simulink model "TLNWithUnrealTestBench"  (R2022b)
settings: Solver=VariableStepAuto  StartTime=0.0  StopTime=scenario.StopTime  FixedStep=0.001  RelTol=1e-8  EnableMultiTasking=on
PostLoadFcn:
  | helperSLTrafficLightNegotiationWithUnrealSetup
values from neighbouring files (symbols this model uses):
  vehSim3D = repmat(         struct(             'Length', 0,             'RearOverhang', 0,             'InitialPos',[0 0 0],             'InitialRot',[0 0 0]),         numVehicles,1)    [helperSLVisionVehicleDetectorSetup.m]
undefined symbols (not defined in the file or in its folder): Curvature, CurvatureDerivative, driving, gray, HeadingAngle, intersectionInfo, LateralOffset, Left, M, matlabshared, N, referencePathInfo, Right, setVelocity, strel, Strength, trafficLightConfig, Ts
libraries: drivingscenarioandsensors x7, visionsinks x4, visiontextngfix x3, sim3dautolib x3, sim3dlib x2, visionstatistics x1, visionmorphops x1, sim3dcameralib x1, helperTrafficLightControllerLib x1, trackingutilitieslib x1, drivinglib x1
CloseFcn:
  | helperSLTrafficLightNegotiationWithUnrealCleanUp
settings Model: Creator=The MathWorks, Inc.  LastModifiedBy=Administrator
settings SolverCC: ZeroCrossAlgorithm=Adaptive  AlgebraicLoopSolver=TrustRegion  PositivePriorityOrder=on  AutoInsertRateTranBlk=on  InsertRTBMode=Always  DecoupledContinuousIntegration=on  MinimalZcImpactIntegration=on  MaxZcPerStep=1
settings DataIOCC: SaveOutput=off  SaveTime=off  ReturnWorkspaceOutputs=off
settings OptimizationCC: DefaultParameterBehavior=Inlined  EnhancedBackFolding=on  PassReuseOutputArgsAs=Individual arguments  ZeroExternalMemoryAtStartup=off  ZeroInternalMemoryAtStartup=off  OptimizeBlockOrder=speed  DifferentSizesBufferReuse=on  OptimizationCustomize=off  EfficientTunableParamExpr=on
settings DebuggingCC: MaskedZcDiagnostic=none  IgnoredZcDiagnostic=none  ParameterPrecisionLossMsg=none  ParameterTunabilityLossMsg=error  UnconnectedInputMsg=warning  UnconnectedOutputMsg=warning  UnconnectedLineMsg=warning  PregeneratedLibrarySubsystemCodeDiagnostic=none  SFMachineParentedDataDiag=warning  ArithmeticOperatorsInVariantConditions=warning
settings HardwareCC: ProdLongLongMode=on
settings ModelReferenceCC: EnableRefExpFcnMdlSchedulingChecks=on
settings SFSimCC: SimUseLocalCustomCode=off  MATLABDynamicMemAlloc=off
settings RTWCC: Description=Embedded Coder  SystemTargetFile=ert.tlc  TemplateMakefile=ert_default_tmf  GenerateReport=on  RTWUseLocalCustomCode=off  LaunchReport=on  DLArmComputeVersion=19.05
settings CodeAppCC: ForceParamTrailComments=on  IgnoreCustomStorageClasses=off  OperatorAnnotations=on  SimulinkDataObjDesc=on  SFDataObjDesc=on  InsertBlockDesc=on
settings ERTTargetCC: TargetLangStandard=C99 (ISO)  GenerateSampleERTMain=on  InlinedParameterPlacement=NonHierarchical  ERTCustomFileTemplate=example_file_process.tlc
settings ConfigComp: CovScope=ReferencedModels  CovIncludeTopModel=off

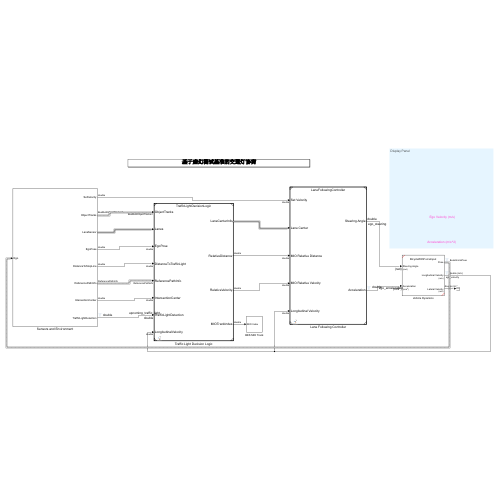
[thumbnail: Simulink's stored preview of the top-level diagram]
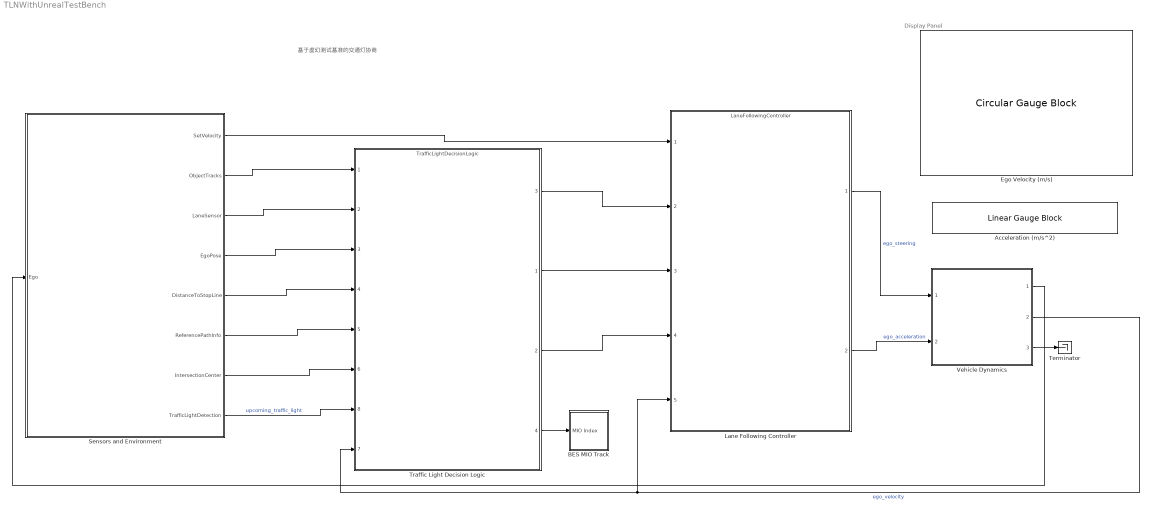
== system TLNWithUnrealTestBench ==
  note: 基于虚幻测试基准的交通灯协商
  note: Display Panel
  Acceleration (m/s^2) : LinearGaugeBlock  LabelPosition=Hide  ScaleMin=-6  ScaleMax=6
  BES MIO Track : Subsystem
  Ego Velocity (m/s) : CircularGaugeBlock  LabelPosition=Hide  ScaleMax=50
  Lane Following Controller : ModelReference  ModelNameDialog=LaneFollowingController.slx  SimulationMode=Normal  ModelReferenceVersion=6.0
  Sensors and Environment : Subsystem
  Terminator : Terminator
  Traffic Light Decision Logic : ModelReference  ModelNameDialog=TrafficLightDecisionLogic  SimulationMode=Normal  ModelReferenceVersion=5.0
      settings: PortSchema="{\"entries\":[{\"content\":{\"sides\":[{\"content\":{\"connectorIds\":[\"In1\",\"In2\",\"In3\",\"In4\",\"In5\",\"In6\",\"In8\",\"In7\"]},\"type\":\"ConnectorPlacement.EquallySpacedRectSide\",\"uuid\":\"80441088-7f88-498e-bd57-56a9591db5ab\"},{\"content\":{\"connectorIds\":[\"Out3\",\"Out1\",\"Out2\",\"Out4\"],\"side\":\"RIGHT\"},\"type\":\"ConnectorPlacement.EquallySpacedRectSide\",\"uuid\":\"71bac071-b53b-4fb3-8fe7-17db6e81a6fe\"},{\"content\":{\"connectorIds\":[],\"side\":\"TOP\"},\"type\":\"ConnectorPlacement.EquallySpacedRectSide\",\"uuid\":\"95fcddf4-1608-4cb5-a6ec-8633d9712dcc\"},{\"content\":{\"connectorIds\":[],\"side\":\"HIDDEN\"},\"type\":\"ConnectorPlacement.EquallySpacedRectSide\",\"uuid\":\"8d5e9fdd-dbcd-4e58-97a7-7da238f3d39d\"}]},\"type\":\"ConnectorPlacement.EquallySpacedConnector\",\"uuid\":\"78ce1c2f-8a23-470e-877e-968badbfaf17\"}],\"packageUris\":[\"http://schema.mathworks.com/mf0/Connector/R2020b\"],\"version\":\"1.0\"}"
  Vehicle Dynamics : Subsystem  ReferencedSubsystem=BicycleWithForceInput
  wires:
  Sensors and Environment/2(ObjectTracks) -> Traffic Light Decision Logic/1
  Sensors and Environment/1(SetVelocity) -> Lane Following Controller/1
  Sensors and Environment/8(TrafficLightDetection) -> Traffic Light Decision Logic/8  "upcoming_traffic_light"
  Vehicle Dynamics/1 -> Sensors and Environment/1(Ego)
  Sensors and Environment/4(EgoPose) -> Traffic Light Decision Logic/3
  Sensors and Environment/3(LaneSensor) -> Traffic Light Decision Logic/2
  Sensors and Environment/5(DistanceToStopLine) -> Traffic Light Decision Logic/4
  Sensors and Environment/6(ReferencePathInfo) -> Traffic Light Decision Logic/5
  Sensors and Environment/7(IntersectionCenter) -> Traffic Light Decision Logic/6
  Lane Following Controller/1 -> Vehicle Dynamics/1  "ego_steering"
  Lane Following Controller/2 -> Vehicle Dynamics/2  "ego_acceleration"
  Traffic Light Decision Logic/3 -> Lane Following Controller/2
  Traffic Light Decision Logic/1 -> Lane Following Controller/3
  Traffic Light Decision Logic/2 -> Lane Following Controller/4
  Traffic Light Decision Logic/4 -> BES MIO Track/1(MIO Index)
  Vehicle Dynamics/2 -> Lane Following Controller/5, Traffic Light Decision Logic/7  "ego_velocity"
  Vehicle Dynamics/3 -> Terminator/1

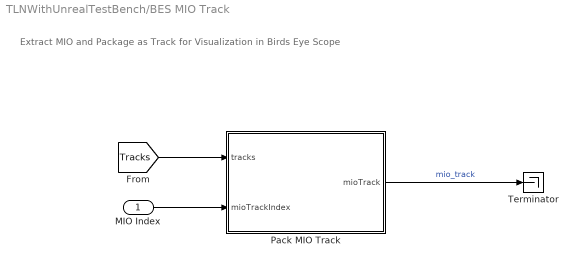
== system TLNWithUnrealTestBench/BES MIO Track ==
  note: Extract MIO and Package as Track for Visualization in Birds Eye Scope
  MIO Index : Inport
  Pack MIO Track : MATLAB Function  TreatAsAtomicUnit=on
  Terminator : Terminator
  wires:
  MIO Index/1 -> Pack MIO Track/2(mioTrackIndex)
  [Tracks] -> Pack MIO Track/1(tracks)
  Pack MIO Track/1(mioTrack) -> Terminator/1  "mio_track"

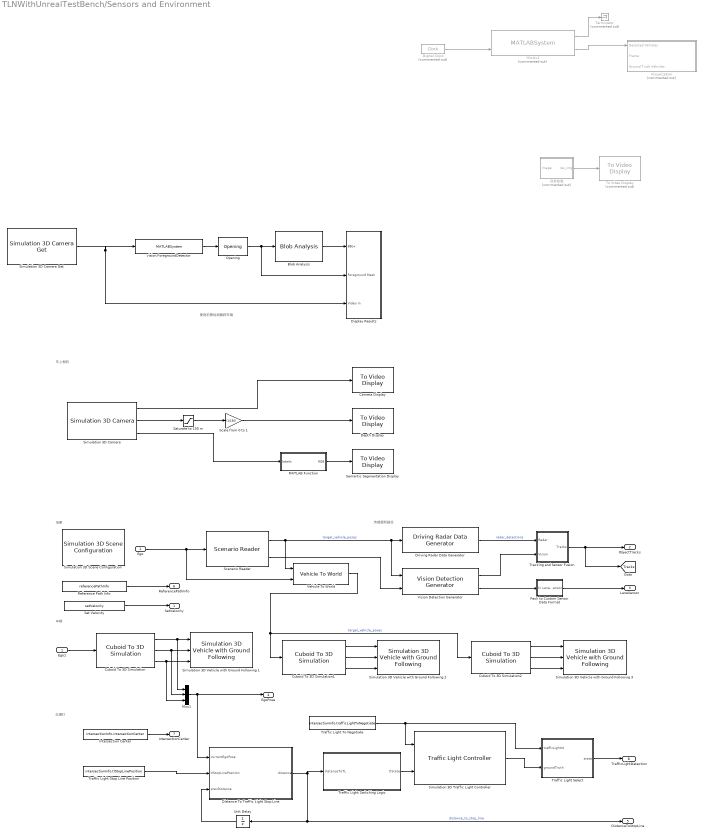
== system TLNWithUnrealTestBench/Sensors and Environment ==
  note: 车上相机
  note: 传感器和融合
  note: 交通灯
  note: 场景
  note: 车辆
  note: 使用前景检测跟踪车辆
  Ego : Inport
  Blob Analysis : visionstatistics/Blob Analysis  Tag=vipblks_row_conv  area=off  centroid=off  bBox=on  majorAxis=off  minorAxis=off  angle=off  eccentricity=off  equivDiameterSq=off  extent=off  perimeter=off  outDT=double  conn=8  isLabel=off  maxBlobs=50  warnIfNumBlobsExceeded=on  isCount=off  useMinArea=on  minArea=150  useMaxArea=off  maxArea=intmax('uint32')  excludeBorderBlob=off  isOutVarDim=on  isFill=on  fillValues=-1  roundingMode=Floor  overflowMode=off  prodOutputMode=Binary point scaling  prodOutputWordLength=32  prodOutputFracLength=16  accumMode=Binary point scaling  accumWordLength=32  accumFracLength=0  outputMode=Binary point scaling  outputWordLength=32  outputFracLength=16  firstCoeffMode=Binary point scaling  firstCoeffWordLength=16  firstCoeffFracLength=14  secondCoeffMode=Binary point scaling  secondCoeffWordLength=32  secondCoeffFracLength=16
  Camera Display : visionsinks/To Video Display  windowSizeMode=Normal  openAtMdlStart=on  fullScreen=off  videoWindowX=536805376  videoWindowY=536805376  saveWindowSize=off  videoWindowWidth=2147483647  videoWindowHeight=2147483647  inputColorFormat=RGB  inputType=Obsolete  imagePorts=One multidimensional signal  OutputDevice=On-screen video monitor  dataOrg=Column-major  isWindowOpen=off
  Cuboid To 3D Simulation : drivingscenarioandsensors/Cuboid To 3D Simulation  SpecifyActorID=off  ActorIDToConvert=1  SimulateUsing=Interpreted execution
  Cuboid To 3D Simulation1 : drivingscenarioandsensors/Cuboid To 3D Simulation  SpecifyActorID=on  ActorIDToConvert=68  SimulateUsing=Interpreted execution
  Cuboid To 3D Simulation2 : drivingscenarioandsensors/Cuboid To 3D Simulation  SpecifyActorID=on  ActorIDToConvert=69  SimulateUsing=Interpreted execution
  Depth Display : visionsinks/To Video Display  windowSizeMode=Normal  openAtMdlStart=on  fullScreen=off  videoWindowX=536805376  videoWindowY=536805376  saveWindowSize=off  videoWindowWidth=1280  videoWindowHeight=720  inputColorFormat=RGB  inputType=Obsolete  imagePorts=One multidimensional signal  OutputDevice=On-screen video monitor  dataOrg=Column-major  isWindowOpen=off
  Digital Clock : DigitalClock  Commented=on  SampleTime=0.1
  Display Results : Subsystem
      settings: RTWMemSecFuncInitTerm=Default  RTWMemSecFuncExecute=Default  RTWMemSecDataConstants=Default  RTWMemSecDataInternal=Default  RTWMemSecDataParameters=Default
  Distance To Traffic Light Stop Line : MATLAB Function  TreatAsAtomicUnit=on  mask{minTLDist=3}
      mask prompts: minTLDist "Minimum distance to traffic light"
  Driving Radar Data Generator : drivingscenarioandsensors/Driving Radar Data Generator  SensorIndex=2  UpdateRate=10  MountingLocation=[ 3.7, 0, 0.2 ]  MountingAngles=[0 0 0]  HasElevation=off  HasRangeRate=on  HasNoise=off  HasFalseAlarms=off  HasOcclusion=on  MaxNumReportsSource=Property  MaxNumReports=50  TargetReportFormat=Clustered detections  DetectionCoordinates=Body  TrackCoordinates=Body  BusNameSource=Property  BusName=BusRadar  AzimuthResolution=4  ElevationResolution=5  RangeResolution=2.5  RangeRateResolution=0.5  AzimuthBiasFraction=0.1  ElevationBiasFraction=0.1  RangeBiasFraction=0.05  RangeRateBiasFraction=0.05  FieldOfView=[ 20, 5 ]  RangeLimits=[ 0, 174 ]  RangeRateLimits=[ -100, 100 ]  DetectionProbability=0.9  FalseAlarmRate=1e-06  ReferenceRange=100  ReferenceRCS=0  CenterFrequency=77e9  FilterInitializationFcn=initcvekf  ConfirmationThreshold=[2 3]  DeletionThreshold=[5 5]  InitialSeedSource=Repeatable  InitialSeed=0  UsedSeed=matlabshared.tracking.internal.SimulinkUtilities.seedManager(gcb)  ProfilesSource=From Scenario Reader block  ProfilesParameters=driving.internal.ActorProfilesRadarParameters  ProfilesExpression=struct('ClassID',0,'Length',4.7,'Width',1.8,'Height',1.4,'OriginOffset',[-1.35 0 0],'RCSPattern',[10 10;10 10],'RCSAzimuthAngles',[-180 180],'RCSElevationAngles',[-90 90])
  Ego1 : InportShadow
  Intersection Center : Constant  Value=intersectionInfo.intersectionCenter  SampleTime=Ts
  MATLAB Function : MATLAB Function  TreatAsAtomicUnit=on
  Mux1 : Mux  Inputs=3
  Opening : visionmorphops/Opening  nhoodsrc=Specify via dialog  strel=strel('square', 3)
  Pack to Custom Sensor Data Format : Subsystem
  Reference Path Info : Constant  Value=referencePathInfo  OutDataTypeStr=Bus: ReferencePathInfo  SampleTime=Ts
  Saturate to 150 m : Saturate  UpperLimit=150  LowerLimit=0
  Scale from 0 to 1 : Gain  Gain=(1/150)
  Scenario Reader : drivingscenarioandsensors/Scenario Reader  ScenarioSource=From workspace  ScenarioFileName=EgoVehicleGoesStraight.mat  ScenarioVariableName=scenario  OutputCoordinateSystem=Vehicle coordinates  EgoVehicleSource=Input port  EgoVehicleActorID=egoVehicle.ActorID  OrientVehiclesOnRoad=on  OutputEgoVehiclePose=off  OutputEgoVehicleState=off  SampleTime=Ts  LaneBoundaryOutput=All lane boundaries  LaneBoundaryDistance=0:0.5:60  LaneBoundaryLocation=Center of lane markings  BusNameSource=Auto  BusName=BusActors  BusNumActorsSource=Scenario  BusNumActors=100  BusName2Source=Auto  BusName2=BusLaneBoundaries  BusNumLaneBoundariesSource=Scenario  BusNumLaneBoundaries=10  BusName3Source=Auto  BusName3=BusEgoActor  BusName4Source=Auto  BusName4=BusEgoState  ShowCoordinateLabels=on  SimulateUsing=Interpreted execution
  Semantic Segmentation Display : visionsinks/To Video Display  windowSizeMode=Normal  openAtMdlStart=on  fullScreen=off  videoWindowX=536805376  videoWindowY=536805376  saveWindowSize=off  videoWindowWidth=1280  videoWindowHeight=720  inputColorFormat=RGB  inputType=Obsolete  imagePorts=One multidimensional signal  OutputDevice=On-screen video monitor  dataOrg=Column-major  isWindowOpen=off
  Set Velocity : Constant  Value=setVelocity
  Simulation 3D Camera : sim3dcameralib/Simulation 3D Camera  Priority=1  sensorTag=Sim3dSensor1  sensorId=1  sensorName=Sim3dSensor1  vehTagList={'EgoVehicle';'Scene Origin';'SimulinkVehicle2';'SimulinkVehicle3'}  vehTag=EgoVehicle  mountLoc=Rearview mirror  offsetFlag=off  tmountOffset=[0, 0, 0]  extTmount=off  rmountOffset=[0, 0, 0]  extRmount=off  FocalLength=[1109, 1109]  OpticalCenter=[640, 360]  ImageSize=[720, 1280]  RadialDistortion=[0, 0]  TangentialDistortion=[0, 0]  SensorSkew=0  DepthOutportEnabled=on  SemanticOutportEnabled=on  TransformOutportEnabled=off  SampleTime=-1  mountPoint=[0.433999985456467 0 1.29999995231628]  mountOrientation=[0 0 0]  aMode=3  ID=1
  Simulation 3D Camera Get : sim3dlib/Simulation 3D Camera Get  Priority=1  sensorTag=Sim3dSensor3  sensorId=3  sensorName=Sim3dSensor3  vehTagList={'EgoVehicle';'Scene Origin';'SimulinkVehicle2';'SimulinkVehicle3'}  vehTag=Scene Origin  mountLoc=Origin  offsetFlag=on  tmountOffset=[-11, 0, 7]  rmountOffset=[0, 15, 180]  HorizontalResolution=1280  VerticalResolution=720  HorizontalFOV=60  SampleTime=-1  mountPoint=[-11 0 7]  mountOrientation=[0 -15 -180]  aMode=5  ID=3
      settings: LibrarySourceBlock=sl3dlib/Simulation 3D/Simulation 3D Camera Get
  Simulation 3D Scene Configuration : sim3dlib/Simulation 3D Scene Configuration  Priority=0  ProjectFormat=Unreal Editor  SceneDesc=US city block  ProjectName=C:\BaiduSyncdisk\matlab\toolbox\shared\sim3d_projects\automotive_project\UE4\WindowsNoEditor\VehicleSimulation.exe  ScenePath=/Game/Maps/USCityBlock  UEProjPath=C:\buffer\AutoVrtlEnv\AutoVrtlEnv.uproject  EnableOpenDRIVE=off  vehTagList={'EgoVehicle';'Scene Origin';'SimulinkVehicle2';'SimulinkVehicle3'}  vehTag=EgoVehicle  OpVisEn=off  Ts=0.1  EnableWindow=on  EnableRemoteAccess=off  EnableWeather=off  SunAltitude=40.0  SunAzimuth=90  clouds=10  wind=1  fog=0  rain=0  EnableGeospatial=off  OriginHeight=200  OriginLatitude=40.744652  OriginLongitude=-73.988864  MapStyle=Aerial  AdditionalAssetIDs=[]  UseAdvancedSunSky=off  SolarTime=11  TimeZone=-5  Day=21  Month=9  Year=2022  UseDaylightSavingTime=on  DSTStartDay=10  DSTStartMonth=3  DSTEndDay=3  DSTEndMonth=11  DSTSwitchHour=2  sensorTag=MainCamera1  sensorId=1  sensorName=MainCamera1  mountLoc=Origin  offsetFlag=off  tmountOffset=[0, 0, 0]  rmountOffset=[0, 0, 0]  HorizontalResolution=1280  VerticalResolution=720  HorizontalFOV=60  mountPoint=[0 0 0]  mountOrientation=[0 0 0]  aMode=3  ID=1  GeoTrigger=Inactive
      settings: AttributesFormatString=SceneDesc = %<SceneDesc>
  Simulation 3D Traffic Light Controller : helperTrafficLightControllerLib/Traffic Light Controller  Priority=-1  helperTrafficLightCheck=0  customScene=0  modeType=State-based  vehTagList={'EgoVehicle';'Scene Origin';'SimulinkVehicle2';'SimulinkVehicle3'}  MsgSize=[1 62]  vehTag=EgoVehicle  trafficLightID=1  greenTime=10  yellowTime=3  redClearanceTime=0  aMode=3  Ts=-1
  Simulation 3D Vehicle with Ground Following 1 : sim3dautolib/Simulation 3D Vehicle with Ground Following  Priority=-1  PassVehMesh=Sedan  MeshPath=/MathWorksSimulation/Vehicles/Muscle/Meshes/SK_MuscleCar.SK_MuscleCar  TrackWidth=1.9  WheelBase=3  WheelRadius=0.35  VehColor=Blue  InitialPos=vehSim3D(1).InitialPos  InitialRot=vehSim3D(1).InitialRot  ActorName=EgoVehicle  SampleTime=-1  ActorType=SimulinkVehicle  ID=C  aMode=3  ActorTag=EgoVehicle  CoordinateScheme=ISO  VehLightsControl=off  HeadlightColor=[ 1, 1, 1 ]  HighBeamIntensity=100000  LowBeamIntensity=60000  HighBeamConeAngle=70  LowBeamConeAngle=70  LeftHeadlightOrientation=[ 0, 0 ]  RightHeadlightOrientation=[ 0, 0 ]  BrakelightIntensity=500  ReverselightIntensity=500  SignallightIntensity=500  SignallightPeriod=1  SignalPulseWidth=50  TransformOutportEnabled=off
      settings: AttributesFormatString=|
      | --------------------------------------
      | ActorName = %<ActorName>
      | PassVehMesh = %<PassVehMesh>
      | VehColor = %<VehColor>
  Simulation 3D Vehicle with Ground Following 2 : sim3dautolib/Simulation 3D Vehicle with Ground Following  Priority=-1  PassVehMesh=Sedan  MeshPath=/MathWorksSimulation/Vehicles/Muscle/Meshes/SK_MuscleCar.SK_MuscleCar  TrackWidth=1.9  WheelBase=3  WheelRadius=0.35  VehColor=Red  InitialPos=vehSim3D(2).InitialPos  InitialRot=vehSim3D(2).InitialRot  ActorName=SimulinkVehicle2  SampleTime=-1  ActorType=SimulinkVehicle  ID=2  aMode=3  ActorTag=SimulinkVehicle2  CoordinateScheme=ISO  VehLightsControl=off  HeadlightColor=[ 1, 1, 1 ]  HighBeamIntensity=100000  LowBeamIntensity=60000  HighBeamConeAngle=70  LowBeamConeAngle=70  LeftHeadlightOrientation=[ 0, 0 ]  RightHeadlightOrientation=[ 0, 0 ]  BrakelightIntensity=500  ReverselightIntensity=500  SignallightIntensity=500  SignallightPeriod=1  SignalPulseWidth=50  TransformOutportEnabled=off
      settings: AttributesFormatString=|
      | --------------------------------------
      | ActorName = %<ActorName>
      | PassVehMesh = %<PassVehMesh>
      | VehColor = %<VehColor>
  Simulation 3D Vehicle with Ground Following 3 : sim3dautolib/Simulation 3D Vehicle with Ground Following  Priority=-1  PassVehMesh=Muscle car  MeshPath=/MathWorksSimulation/Vehicles/Muscle/Meshes/SK_MuscleCar.SK_MuscleCar  TrackWidth=1.9  WheelBase=3  WheelRadius=0.35  VehColor=Black  InitialPos=vehSim3D(3).InitialPos  InitialRot=vehSim3D(3).InitialRot  ActorName=SimulinkVehicle3  SampleTime=-1  ActorType=SimulinkVehicle  ID=3  aMode=3  ActorTag=SimulinkVehicle3  CoordinateScheme=ISO  VehLightsControl=off  HeadlightColor=[ 1, 1, 1 ]  HighBeamIntensity=100000  LowBeamIntensity=60000  HighBeamConeAngle=70  LowBeamConeAngle=70  LeftHeadlightOrientation=[ 0, 0 ]  RightHeadlightOrientation=[ 0, 0 ]  BrakelightIntensity=500  ReverselightIntensity=500  SignallightIntensity=500  SignallightPeriod=1  SignalPulseWidth=50  TransformOutportEnabled=off
      settings: AttributesFormatString=|
      | --------------------------------------
      | ActorName = %<ActorName>
      | PassVehMesh = %<PassVehMesh>
      | VehColor = %<VehColor>
  Terminator : Terminator  Commented=on
  To Video Display : visionsinks/To Video Display  Commented=on  windowSizeMode=Normal  openAtMdlStart=on  fullScreen=off  videoWindowX=367  videoWindowY=270  saveWindowSize=off  videoWindowWidth=1280  videoWindowHeight=720  inputColorFormat=RGB  inputType=Obsolete  imagePorts=One multidimensional signal  OutputDevice=On-screen video monitor  dataOrg=Column-major  isWindowOpen=off
  Tracking and Sensor Fusion : Subsystem  TreatAsAtomicUnit=on
      settings: RTWFileNameOpts=Use function name
  Traffic Light Select : MATLAB Function  TreatAsAtomicUnit=on
  Traffic Light Stop Line Position : Constant  Value=intersectionInfo.tlStopLinePosition  OutDataTypeStr=double
  Traffic Light Switching Logic : Stateflow chart  TreatAsAtomicUnit=on  SystemSampleTime=Ts  mask{tlConfig=trafficLightConfig}
      mask prompts: tlConfig "Configuration Params"
  Traffic Light To Negotiate : Constant  Value=intersectionInfo.trafficLightToNegotiate
  Unit Delay : UnitDelay  InitialCondition=100  SampleTime=-1  HasFrameUpgradeWarning=on
  Vehicle To World : drivingscenarioandsensors/Vehicle To World  BusNameSource=Auto  BusName=BusVehicleToWorldActors  SimulateUsing=Interpreted execution
  Vision Detection Generator : drivingscenarioandsensors/Vision Detection Generator  SensorIndex=1  DetectorOutput=Lanes and objects  UpdateInterval=0.1  LaneUpdateInterval=0.1  SensorLocation=[ 1.9, 0 ]  Height=1.1  Yaw=0  Pitch=1  Roll=0  BusNameSource=Property  BusName=BusVision  BusName2Source=Property  BusName2=BusLanes  MaxNumDetectionsSource=Property  MaxNumDetections=20  MaxNumLanesSource=Property  MaxNumLanes=2  DetectionCoordinates=Ego Cartesian  SimulateUsing=Interpreted execution  MaxRange=150  BoundingBoxAccuracy=5  ProcessNoiseIntensity=5  MaxSpeed=50  MaxAllowedOcclusion=0.5  MinObjectImageSize=[ 10, 10 ]  DetectionProbability=0.9  FalsePositivesPerImage=0.1  MinLaneImageSize=[ 20, 3 ]  LaneBoundaryAccuracy=3  HasNoise=on  InitialSeedSource=Repeatable  InitialSeed=0  UsedSeed=driving.internal.SimulinkUtilities.seedManager(gcb)  ActorProfilesSource=From Scenario Reader block  ActorProfilesParameters=driving.internal.ActorProfilesParameters  ActorProfilesExpression=struct( 'ClassID', 0, 'Length', 4.7, 'Width', 1.8, 'Height', 1.4, 'OriginOffset', [ -1.35, 0, 0 ] )  Intrinsics=driving.internal.cameraIntrinsics('FocalLength',[ 800,800 ])
  Visualization : Subsystem  Commented=on
  YOLOv2 : MATLABSystem  Commented=on  System=HelperVisionVehicleDetector  EnableDisplay=off  Detector=VehicleDetector.YOLOv2  Camera=frame  SimulateUsing=Interpreted execution
      mask Type: HelperVisionVehicleDetector
      mask Display:
      | disp('HelperVisionVehicleDetector');
      | port_label('input',1,'frame');
      | port_label('input',2,'t');
      | port_label('output',1,'vehicles');
      | port_label('output',2,'detectionsInfo');
  vision.ForegroundDetector : MATLABSystem  System=vision.ForegroundDetector  NumGaussians=3  MinimumBackgroundRatio=0.7  InitialVariance=Auto  AdaptLearningRate=on  NumTrainingFrames=50  LearningRate=0.005  SimulateUsing=Interpreted execution
      mask Type: vision.ForegroundDetector
      mask Display:
      | disp('ForegroundDetector');
      | port_label('output',1,'fgMask');
  目标检测 : MATLAB Function  Commented=on  TreatAsAtomicUnit=on
  SetVelocity : Outport
  ObjectTracks : Outport  Port=2
  LaneSensor : Outport  Port=3  VectorParamsAs1DForOutWhenUnconnected=off
  EgoPose : Outport  Port=4
  DistanceToStopLine : Outport  Port=5
  ReferencePathInfo : Outport  Port=6
  IntersectionCenter : Outport  Port=7
  TrafficLightDetection : Outport  Port=8  SampleTime=Ts
  tag scope: Tracks=global
  wires:
  Scenario Reader/1 -> Vehicle To World/1, Driving Radar Data Generator/1, Vision Detection Generator/1  "target_vehicle_poses"
  Cuboid To 3D Simulation1/3 -> Simulation 3D Vehicle with Ground Following 2/3
  Cuboid To 3D Simulation1/2 -> Simulation 3D Vehicle with Ground Following 2/2
  Cuboid To 3D Simulation2/2 -> Simulation 3D Vehicle with Ground Following 3/2
  Cuboid To 3D Simulation2/3 -> Simulation 3D Vehicle with Ground Following 3/3
  Vehicle To World/1 -> Cuboid To 3D Simulation1/1, Cuboid To 3D Simulation2/1  "target_vehicle_poses"
  Cuboid To 3D Simulation1/1 -> Simulation 3D Vehicle with Ground Following 2/1
  Cuboid To 3D Simulation2/1 -> Simulation 3D Vehicle with Ground Following 3/1
  Scenario Reader/2 -> Vision Detection Generator/2
  Driving Radar Data Generator/1 -> Tracking and Sensor Fusion/1(Radar)  "radar_detections"
  Vision Detection Generator/1 -> Tracking and Sensor Fusion/2(Vision)
  Tracking and Sensor Fusion/1(Tracks) -> [Tracks], ObjectTracks/1
  Vision Detection Generator/2 -> Pack to Custom Sensor Data Format/1(In)
  Pack to Custom Sensor Data Format/1(LaneSensor) -> LaneSensor/1
  Traffic Light Switching Logic/1(tlState) -> Simulation 3D Traffic Light Controller/2
  Traffic Light Stop Line Position/1 -> Distance To Traffic Light Stop Line/2(tlStopLinePosition)
  Simulation 3D Traffic Light Controller/1 -> Traffic Light Select/2(groundTruth)
  Traffic Light Select/1(state) -> TrafficLightDetection/1
  Ego/1 -> Scenario Reader/1, Vehicle To World/2
  Ego1/1 -> Cuboid To 3D Simulation/1
  Cuboid To 3D Simulation/2 -> Mux1/2, Simulation 3D Vehicle with Ground Following 1/2
  Cuboid To 3D Simulation/1 -> Mux1/1, Simulation 3D Vehicle with Ground Following 1/1
  Cuboid To 3D Simulation/3 -> Mux1/3, Simulation 3D Vehicle with Ground Following 1/3
  Distance To Traffic Light Stop Line/1(distance) -> Traffic Light Switching Logic/1(distanceToTL), Unit Delay/1, DistanceToStopLine/1  "distance_to_stop_line"
  Mux1/1 -> EgoPose/1, Distance To Traffic Light Stop Line/1(currentEgoPose)
  Traffic Light To Negotiate/1 -> Simulation 3D Traffic Light Controller/1, Traffic Light Select/1(trafficLightId)
  Intersection Center/1 -> IntersectionCenter/1
  Unit Delay/1 -> Distance To Traffic Light Stop Line/3(prevDistance)
  Reference Path Info/1 -> ReferencePathInfo/1
  Set Velocity/1 -> SetVelocity/1
  Simulation 3D Camera/1 -> Camera Display/1
  Scale from 0 to 1/1 -> Depth Display/1
  Saturate to 150 m/1 -> Scale from 0 to 1/1
  MATLAB Function/1(RGB) -> Semantic Segmentation Display/1
  Simulation 3D Camera/3 -> MATLAB Function/1(labels)
  Simulation 3D Camera/2 -> Saturate to 150 m/1
  目标检测/1(res_img) -> To Video Display/1
  Digital Clock/1 -> YOLOv2/2
  YOLOv2/2 -> Visualization/1(Detected Vehicles)
  YOLOv2/1 -> Terminator/1
  vision.ForegroundDetector/1 -> Opening/1
  Blob Analysis/1 -> Display Results/1(BBox)
  Opening/1 -> Blob Analysis/1, Display Results/2(Foreground Mask)
  Simulation 3D Camera Get/1 -> Display Results/3(Video In), vision.ForegroundDetector/1

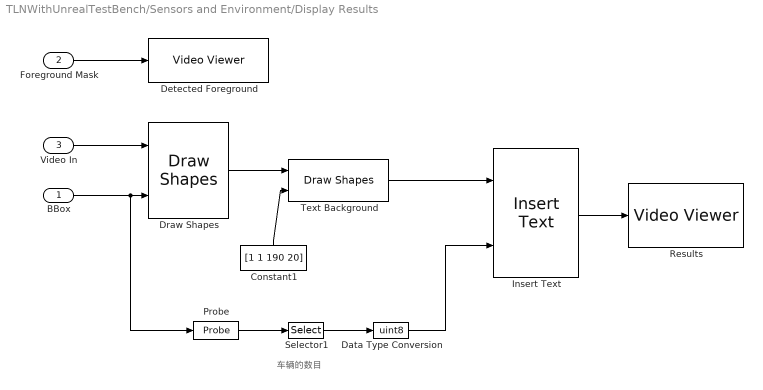
== system TLNWithUnrealTestBench/Sensors and Environment/Display Results ==
  note: 车辆的数目
  BBox : Inport
  Foreground Mask : Inport  Port=2
  Video In : Inport  Port=3
  Constant1 : Constant  Value=[1 1 190 20]  OutDataTypeStr=uint16
  Data Type Conversion : DataTypeConversion  OutDataTypeStr=uint8  SaturateOnIntegerOverflow=off  RndMeth=Floor
  Detected Foreground : VideoViewer  colormapValue=gray(256)  FigPos=[22 517 623 421]  trueSizedOnce=on
  Draw Shapes : visiontextngfix/Draw Shapes  shape=Rectangles  fill=off  lineWidth=1  fillClrSource=Specify via dialog  display=User-specified value  intensity=200  color=[0 1 0]  opacity=0.6  viewport=Entire image  antialiasing=off  inType=Obsolete  imagePorts=One multidimensional signal  roundingMode=Floor  overflowMode=off  memoryMode=Specify word length  memoryWordLength=16  prodOutputMode=Binary point scaling  prodOutputWordLength=32  prodOutputFracLength=14  memoryFracLength=15
  Insert Text : visiontextngfix/Insert Text  inputType=Obsolete  theText='Number of Cars: %d'  getTextLocFrom=Specify via dialog  textLoc=[1 1]  getTextColorFrom=Specify via dialog  textColor=[1 1 1]  getTextIntensityFrom=Specify via dialog  textIntensity=1  getTextOpacityFrom=Specify via dialog  textOpacity=1.0  dummyVar2=0  dummyVar3=0  dummyVar4=0  imagePorts=One multidimensional signal  isInputTransposed=off  fontFace=LucidaSansRegular  dummyVar1=0  blockFontSize=16  antiAliased=on
  Probe : Probe  ProbeWidth=off  ProbeSampleTime=off  ProbeComplexSignal=off  ProbeSignalDimensions=on  ProbeWidthDataType=uint8
  Results : VideoViewer  colormapValue=gray(256)  FigPos=[616 517 637 427]  trueSizedOnce=on
  Selector1 : Selector  NumberOfDimensions=2  InputPortWidth=3  IndexOptions=Index vector (dialog),Index vector (dialog)  Indices=1,1  OutputSizes=99,1
  Text Background : visiontextngfix/Draw Shapes  shape=Rectangles  fill=on  lineWidth=1  fillClrSource=Specify via dialog  display=User-specified value  intensity=200  color=[0 0 0]  opacity=1  viewport=Entire image  antialiasing=off  inType=Obsolete  imagePorts=One multidimensional signal  roundingMode=Floor  overflowMode=off  memoryMode=Specify word length  memoryWordLength=16  prodOutputMode=Binary point scaling  prodOutputWordLength=32  prodOutputFracLength=14  memoryFracLength=14
  wires:
  Foreground Mask/1 -> Detected Foreground/1
  Data Type Conversion/1 -> Insert Text/2
  Selector1/1 -> Data Type Conversion/1
  Probe/1 -> Selector1/1
  Insert Text/1 -> Results/1
  Text Background/1 -> Insert Text/1
  Draw Shapes/1 -> Text Background/1
  Constant1/1 -> Text Background/2
  BBox/1 -> Probe/1, Draw Shapes/2
  Video In/1 -> Draw Shapes/1

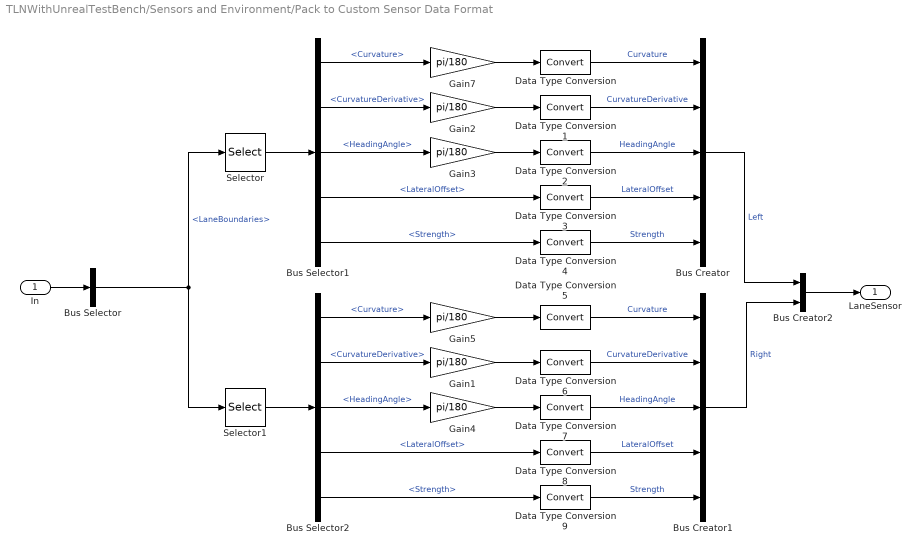
== system TLNWithUnrealTestBench/Sensors and Environment/Pack to Custom Sensor Data Format ==
  In : Inport
  Bus Creator : BusCreator  Inputs=Curvature,CurvatureDerivative,HeadingAngle,LateralOffset,Strength  OutDataTypeStr=Bus: LaneSensorBoundaries
  Bus Creator1 : BusCreator  Inputs=Curvature,CurvatureDerivative,HeadingAngle,LateralOffset,Strength  OutDataTypeStr=Bus: LaneSensorBoundaries
  Bus Creator2 : BusCreator  Inputs=Left,Right  OutDataTypeStr=Bus: LaneSensor
  Bus Selector : BusSelector  OutputSignals=LaneBoundaries
  Bus Selector1 : BusSelector  OutputSignals=Curvature,CurvatureDerivative,HeadingAngle,LateralOffset,Strength
  Bus Selector2 : BusSelector  OutputSignals=Curvature,CurvatureDerivative,HeadingAngle,LateralOffset,Strength
  Data Type Conversion{,1..9} (10 alike) : DataTypeConversion  SaturateOnIntegerOverflow=off  RndMeth=Floor
  Gain{1..5,7} (6 alike) : Gain  Gain=pi/180
  Selector : Selector  InputPortWidth=2  IndexOptions=Index vector (dialog)  Indices=1  OutputSizes=1
  Selector1 : Selector  InputPortWidth=2  IndexOptions=Index vector (dialog)  Indices=2  OutputSizes=1
  LaneSensor : Outport  VectorParamsAs1DForOutWhenUnconnected=off
  wires:
  In/1 -> Bus Selector/1
  Bus Selector/1 -> Selector/1, Selector1/1  "<LaneBoundaries>"
  Selector/1 -> Bus Selector1/1
  Bus Selector1/2 -> Gain2/1  "<CurvatureDerivative>"
  Bus Selector1/1 -> Gain7/1  "<Curvature>"
  Bus Selector1/3 -> Gain3/1  "<HeadingAngle>"
  Gain7/1 -> Data Type Conversion/1
  Gain2/1 -> Data Type Conversion1/1
  Gain3/1 -> Data Type Conversion2/1
  Bus Selector1/4 -> Data Type Conversion3/1  "<LateralOffset>"
  Bus Selector1/5 -> Data Type Conversion4/1  "<Strength>"
  Data Type Conversion/1 -> Bus Creator/1  "Curvature"
  Data Type Conversion1/1 -> Bus Creator/2  "CurvatureDerivative"
  Data Type Conversion2/1 -> Bus Creator/3  "HeadingAngle"
  Data Type Conversion3/1 -> Bus Creator/4  "LateralOffset"
  Data Type Conversion4/1 -> Bus Creator/5  "Strength"
  Data Type Conversion9/1 -> Bus Creator1/5  "Strength"
  Data Type Conversion6/1 -> Bus Creator1/2  "CurvatureDerivative"
  Data Type Conversion7/1 -> Bus Creator1/3  "HeadingAngle"
  Data Type Conversion8/1 -> Bus Creator1/4  "LateralOffset"
  Data Type Conversion5/1 -> Bus Creator1/1  "Curvature"
  Bus Selector2/1 -> Gain5/1  "<Curvature>"
  Selector1/1 -> Bus Selector2/1
  Bus Selector2/4 -> Data Type Conversion8/1  "<LateralOffset>"
  Bus Selector2/5 -> Data Type Conversion9/1  "<Strength>"
  Bus Selector2/2 -> Gain1/1  "<CurvatureDerivative>"
  Gain4/1 -> Data Type Conversion7/1
  Gain5/1 -> Data Type Conversion5/1
  Gain1/1 -> Data Type Conversion6/1
  Bus Selector2/3 -> Gain4/1  "<HeadingAngle>"
  Bus Creator2/1 -> LaneSensor/1
  Bus Creator/1 -> Bus Creator2/1  "Left"
  Bus Creator1/1 -> Bus Creator2/2  "Right"

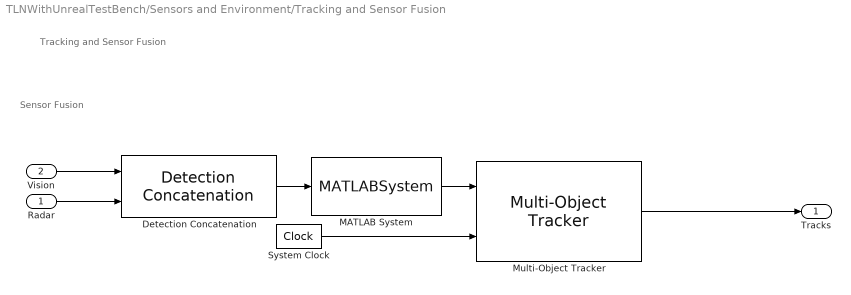
== system TLNWithUnrealTestBench/Sensors and Environment/Tracking and Sensor Fusion ==
  note: Tracking and Sensor Fusion
  note: Sensor Fusion
  Radar : Inport  OutDataTypeStr=Bus: BusRadar  PortDimensions=[1 1]  BusOutputAsStruct=on
  Vision : Inport  Port=2  OutDataTypeStr=Bus: BusVision  PortDimensions=[1 1]  BusOutputAsStruct=on
  Detection Concatenation : trackingutilitieslib/Detection Concatenation  NumInputs=2  BusNameSource=Auto  BusName=BusDetectionConcatenation  SimulateUsing=Interpreted execution
  MATLAB System : MATLABSystem  System=helperVehicleSize  VehicleSize=vehicleLength  BusNameSource=Auto  BusName=BusVehicleSizeDetections  SimulateUsing=Interpreted execution
      mask Type: helperVehicleSize
      mask Display:
      | disp('helperVehicleSize');
      | port_label('input',1,'In');
      | port_label('output',1,'Out');
  Multi-Object Tracker : drivinglib/Multi-Object Tracker  TrackerIndex=uint32( 0 )  FilterInitializationFcn=initcvekf  AssignmentThreshold=assigThresh  ConfirmationThreshold=[ M, N ]  DeletionThreshold=[ 5, 5 ]  MaxNumTracks=numTracks  MaxNumSensors=numSensors  OOSMHandling=Terminate  StateParametersSimulink=struct  HasStateParametersInput=off  TimeInputSource=Input port  HasCostMatrixInput=off  HasDetectableTrackIDsInput=off  BusNameSource=Property  BusName=BusMultiObjectTracker1  TentativeTracksOutputPort=off  AllTracksOutputPort=off  SimulateUsing=Interpreted execution
  System Clock : DigitalClock  SampleTime=Ts
  Tracks : Outport  OutDataTypeStr=Bus:BusMultiObjectTracker1  PortDimensions=[1 1]  VectorParamsAs1DForOutWhenUnconnected=off  BusOutputAsStruct=on
  wires:
  Detection Concatenation/1 -> MATLAB System/1
  Multi-Object Tracker/1 -> Tracks/1
  Radar/1 -> Detection Concatenation/2
  System Clock/1 -> Multi-Object Tracker/2
  Vision/1 -> Detection Concatenation/1
  MATLAB System/1 -> Multi-Object Tracker/1

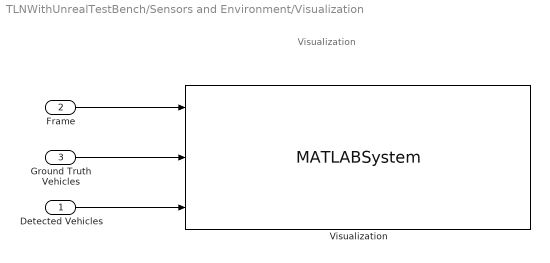
== system TLNWithUnrealTestBench/Sensors and Environment/Visualization ==
  note: Visualization
  Detected Vehicles : Inport
  Frame : Inport  Port=2
  Ground Truth Vehicles : Inport  Port=3
  Visualization : MATLABSystem  System=HelperVisualizeVehicles  EnableTruthDisplay=off  Camera=camera
      mask Type: HelperVisualizeVehicles
      mask Display:
      | disp('HelperVisualizeVehicles');
      | port_label('input',1,'frame');
      | port_label('input',2,'groundTruthVehicles');
      | port_label('input',3,'detectedVehicles');
  wires:
  Frame/1 -> Visualization/1
  Ground Truth Vehicles/1 -> Visualization/2
  Detected Vehicles/1 -> Visualization/3

== matlab function TLNWithUnrealTestBench/Sensors and Environment/MATLAB Function ==
  data: labels input; RGB output
function RGB = sim3dlabel2rgb(labels)
% Convert semantic segmentation map captured during 3D simulation to RGB
% color image.

% Declare label2rgb function.
coder.extrinsic('label2rgb');

% Preallocate memory for RGB matrix.
RGB = coder.nullcopy(zeros(size(labels,1),size(labels,2),3,class(labels)));

% Define colormap using 3D simulation label IDs.
cmap = sim3dColormap;

% Convert labels to RGB color image.
RGB = label2rgb(labels, cmap);

== matlab function TLNWithUnrealTestBench/Sensors and Environment/Traffic Light Select ==
  data: trafficLightId input; groundTruth input; state output
function state   = trafficLightSelect(trafficLightId, groundTruth)
% trafficLightSelect 选择在智能车控制下的交通灯并输出其状态

% US City Block 场景中有30个交通灯，所以有效的交通灯ID是在1到30之间。
if(trafficLightId >=1 && trafficLightId <= 30)
    % 从真实信息中获得即将到来的交通灯状态upcomingTrafficLight
    state = groundTruth(trafficLightId, 2);
else
    % 如果即将到来交通灯ID是0，那么将交通灯状态设置为-1，表示没有检测到交通灯。
    state = -1;
end

end

== matlab function TLNWithUnrealTestBench/BES MIO Track/Pack MIO Track ==
  data: tracks input; mioTrack output Bus: BusMultiObjectTracker1; mioTrackIndex input
function mioTrack = fcn(tracks, mioTrackIndex)
% Extract MIO track and package for visualization in Birds Eye Scope

mioTrack = tracks;

if mioTrackIndex > 0
    % First track represents MIO
    mioTrack.NumTracks = 1;
    mioTrack.Tracks(1) = tracks.Tracks(mioTrackIndex);
else
    % No valid MIO track
    mioTrack.NumTracks = 0;
end

== matlab function TLNWithUnrealTestBench/Sensors and Environment/目标检测 ==
  data: image input; res_img output
function res_img = car_detection(image)
% simulink代码生成的过程中，有些函数是不支持内部代码生成的，需要将其定义为外部函数，使用coder.extrinsic声明一下即可
% 参考：workspace\demo\Examples\R2022b\driving\PerceptionBasedParkingSpotsDetectionUsingUnrealEngineExample
% open('C:\BaiduSyncdisk\workspace\demo\Examples\R2022b\driving\PerceptionBasedParkingSpotsDetectionUsingUnrealEngineExample\ParkingLaneMarkingsDetection.slx');

% coder.extrinsic('helper_car_detection')
% helper_car_detection(image);

res_img = image;

== matlab function TLNWithUnrealTestBench/Sensors and Environment/Distance To Traffic Light Stop Line ==
  data: currentEgoPose input; tlStopLinePosition input; prevDistance input; distance output; minTLDist parameter
function distance   = distanceToTrafficLight(currentEgoPose, tlStopLinePosition, prevDistance, minTLDist)

%distanceToTrafficLight Compute distance to upcoming traffic light.

distance = ...
    helperSLComputeDistanceToTrafficLight(tlStopLinePosition, ...
    currentEgoPose, prevDistance, minTLDist);

== stateflow chart TLNWithUnrealTestBench/Sensors and Environment/Traffic Light Switching Logic ==
  state ENTER
    entry:
    tlState =  tlConfig.initialState;
  state GREEN_STATE
    entry:
    tlState = Green;
  state YELLOW_STATE
    entry:
    tlState = Yellow;
  state RED_STATE
    entry:
    tlState = Red;
  (default) -> ENTER
  ENTER -> (junction 126) [order 1]
  (junction 126) -> RED_STATE : [[tlConfig.initialState == Red]]
  ENTER -> GREEN_STATE [order 2] : [[tlConfig.initialState == Green]]
  (junction 114) -> RED_STATE
  RED_STATE -> (junction 118)
  (junction 124) -> YELLOW_STATE
  YELLOW_STATE -> (junction 116) : after(1,sec)
  (junction 120) -> GREEN_STATE
  GREEN_STATE -> (junction 122)
  (junction 118) -> (junction 120) : [distanceToTL < tlConfig.stateChangeDistance ...
      | && tlConfig.changeState == Green]
  (junction 122) -> (junction 124) : [distanceToTL < tlConfig.stateChangeDistance ...
      | && tlConfig.changeState == Red]
  (junction 116) -> (junction 114)
  data: tlState output =  tlConfig.initialState; Green constant double =2; Red constant double =0; Yellow constant double =1; distanceToTL input; tlConfig parameter
